simulink model "MicroFSMPCCLACPU1"  (R2024a)
settings: Solver=FixedStepAuto  StartTime=0.0  StopTime=Inf  RelTol=1e-3  EnableMultiTasking=on
values from neighbouring files (symbols this model uses):
  ar = single(round(1/10,3))    [Para_Motor_Micro.m]
  PI_params = mcb.internal.SetControllerParameters(pmsm,inverter,SI_System,T_pwm,Ts,Ts_speed)    [Para_Motor_Micro.m]
  Tabf = round(Tab',3)    [Para_Motor_Micro.m]
  target = mcb_SetProcessorDetails('F28379D',PWM_frequency)    [Para_Motor_Micro.m]
  Ts = T_pwm    (= 3e-05)    [Para_Motor_Micro.m]
  Ts_com = 2*1*Ts    (= 6e-05)    [Para_Motor_Micro.m]
undefined symbols (not defined in the file or in its folder): C28x, codertarget, CPU1, CPU2, Down, dyV, gmax, GPTRIP1SEL, GPTRIP2SEL, inverter, Ls, PWM_Counter_PeriodVel, R, Tab, Tv, Tvz, TZ1, TZ2, ud, Up
libraries: mcbcontrolslib x28, c2802xlib x18, c2837xDlib x13, dsparch4 x6, eeTransforms x5, slpidlib x4, mcbpositiondecoderlib x3, simulink x2, c2806xlib x1, spsabctoAlphaBetaZeroLib x1, c280xlib x1, c2000lib x1
(part 1 of 8)
settings Model: ExtModeTrigDuration=8  Creator=axel_  LastModifiedBy=axel_
settings SolverCC: AutoInsertRateTranBlk=on
settings OptimizationCC: DefaultParameterBehavior=Inlined  DefaultUnderspecifiedDataType=single  EnhancedBackFolding=on  PassReuseOutputArgsAs=Individual arguments  MaxStackSize=1024  OptimizeBlockOrder=speed  DifferentSizesBufferReuse=on  OptimizationCustomize=off  DenormalBehavior=FlushToZero  EfficientTunableParamExpr=on
settings DebuggingCC: MultiTaskDSMMsg=none  ParameterPrecisionLossMsg=none  ParameterTunabilityLossMsg=error
settings HardwareCC: ProdBitPerChar=16  ProdBitPerInt=16  ProdBitPerPointer=32  ProdBitPerSizeT=32  ProdBitPerPtrDiffT=32  ProdLargestAtomicInteger=Integer  ProdLargestAtomicFloat=None  ProdWordSize=16  ProdHWDeviceType=Texas Instruments->C2000
settings ModelReferenceCC: ModelReferenceNumInstancesAllowed=Single
settings SFSimCC: MATLABDynamicMemAlloc=off
settings RTWCC: Description=Embedded Coder  SystemTargetFile=ert.tlc  HardwareBoard=TI Delfino F2837xD  TemplateMakefile=ert_default_tmf  Toolchain=Texas Instruments Code Composer Studio (C2000)  GPUComputeCapability=3.5
settings CodeAppCC: ForceParamTrailComments=on  IgnoreCustomStorageClasses=off  OperatorAnnotations=on  SimulinkDataObjDesc=on  SFDataObjDesc=on  InsertBlockDesc=on
settings ERTTargetCC: CodeReplacementLibrary=TI C28x  ExtModeTransport=4  ExtModeStaticAlloc=on  ExtModeAutomaticAllocSize=off  ExtModeStaticAllocSize=10000  ExtModeMexFile=ext_xcp  ExtModeIntrfLevel=Level2 - Open  InlinedParameterPlacement=NonHierarchical

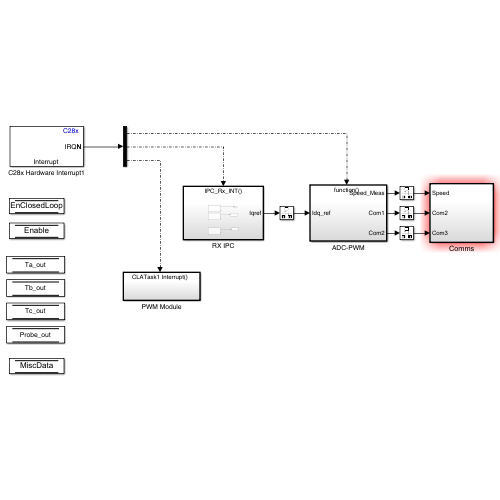
[thumbnail: Simulink's stored preview of the top-level diagram]
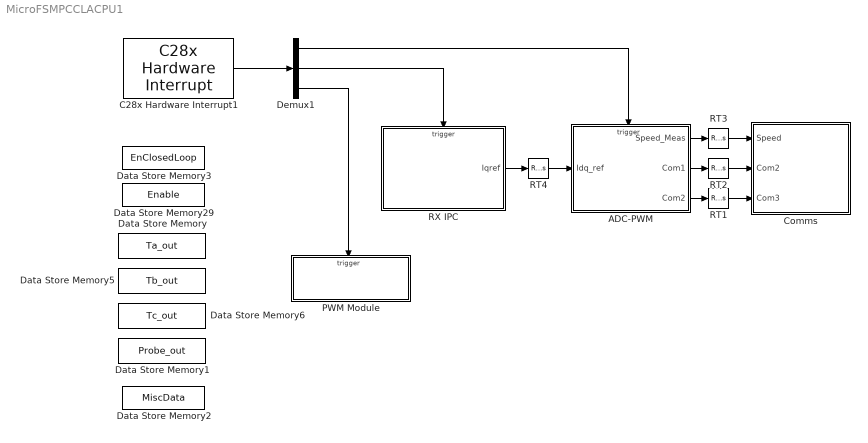
== system MicroFSMPCCLACPU1 ==
  "ADC-PWM " : Subsystem  TreatAsAtomicUnit=on
  C28x Hardware Interrupt1 : c2000lib/Scheduling/C28x Hardware Interrupt  irqnumbers=[1 1 11 ]  pienumbers=[1 15 1 ]  irqpriorities="[30 40  27 ]"  irqpreempts="[1   0  1 ]"  showinput=off  dspchiptype=C280X
  Comms : Subsystem  TreatAsAtomicUnit=on  SystemSampleTime=Ts_com
  Data Store Memory2 : DataStoreMemory  DataStoreName=MiscData  InitialValue=2*pi*0.1296+0.05247  ShowAdditionalParam=off  OutDataTypeStr=single
  Data Store Memory29 : DataStoreMemory  DataStoreName=Enable  ShowAdditionalParam=off  OutDataTypeStr=boolean
  Data Store Memory3 : DataStoreMemory  DataStoreName=EnClosedLoop  ShowAdditionalParam=off  OutDataTypeStr=boolean
  Data Store Memory : DataStoreMemory  DataStoreName=Ta_out  ReadBeforeWriteMsg=warning  WriteAfterWriteMsg=warning  WriteAfterReadMsg=warning  ShowAdditionalParam=off  OutDataTypeStr=single
  Data Store Memory1 : DataStoreMemory  DataStoreName=Probe_out  ReadBeforeWriteMsg=warning  WriteAfterWriteMsg=warning  WriteAfterReadMsg=warning  ShowAdditionalParam=off  OutDataTypeStr=single
  Data Store Memory5 : DataStoreMemory  DataStoreName=Tb_out  ReadBeforeWriteMsg=warning  WriteAfterWriteMsg=warning  WriteAfterReadMsg=warning  ShowAdditionalParam=off  OutDataTypeStr=single
  Data Store Memory6 : DataStoreMemory  DataStoreName=Tc_out  ReadBeforeWriteMsg=warning  WriteAfterWriteMsg=warning  WriteAfterReadMsg=warning  ShowAdditionalParam=off  OutDataTypeStr=single
  Demux1 : Demux  Outputs=3
  PWM Module : Subsystem  TreatAsAtomicUnit=on
  RT{1..4} (4 alike) : RateTransition  Deterministic=off
  RX IPC : Subsystem
  wires:
  C28x Hardware Interrupt1/1 -> Demux1/1
  Demux1/1 -> "ADC-PWM "/Trigger
  "ADC-PWM "/1(Speed_Meas) -> RT3/1
  "ADC-PWM "/2(Com1) -> RT2/1
  "ADC-PWM "/3(Com2) -> RT1/1
  RT3/1 -> Comms/1(Speed)
  RT2/1 -> Comms/2(Com2)
  RT1/1 -> Comms/3(Com3)
  RX IPC/1(Iqref) -> RT4/1
  Demux1/2 -> RX IPC/Trigger
  Demux1/3 -> PWM Module/Trigger
  RT4/1 -> "ADC-PWM "/1(Idq_ref)

== system MicroFSMPCCLACPU1/ADC-PWM  ==
  Idq_ref : Inport
  function : TriggerPort  TriggerType=function-call  VariantControl=Variant  OutputDataType=int8
  Constant : Constant
  Control_System : Subsystem  TreatAsAtomicUnit=on
  Demux1 : Demux  Outputs=2
  Demux2 : Demux  Outputs=2
  Digital Output2 : c2837xDlib/Digital Output  GPIO_Number=GPIO32~GPIO39  GPIO_Bit0=off  GPIO_BIT0_Toggle=on  GPIO_Bit1=off  GPIO_BIT1_Toggle=off  GPIO_Bit2=off  GPIO_BIT2_Toggle=off  GPIO_Bit3=off  GPIO_BIT3_Toggle=off  GPIO_Bit4=off  GPIO_BIT4_Toggle=off  GPIO_Bit5=off  GPIO_BIT5_Toggle=off  GPIO_Bit6=off  GPIO_BIT6_Toggle=off  GPIO_Bit7=on  GPIO_BIT7_Toggle=on
  Mesurments : Subsystem
  Speed_Meas : Outport
  Com1 : Outport  Port=2
  Com2 : Outport  Port=3
  wires:
  Idq_ref/1 -> Control_System/3(Tref)
  Mesurments/1(I) -> Control_System/1(Imesure)
  Mesurments/5(Thetae) -> Control_System/4(PosE)
  Mesurments/2(Voltage Bus) -> Control_System/2(Voltage Bus)
  Control_System/2(Debug control 2) -> Demux1/1
  Constant/1 -> Digital Output2/1
  Mesurments/6(Speedencoder) -> Speed_Meas/1, Control_System/5(Speed)
  Control_System/1(Debug control) -> Demux2/1
  Demux2/2 -> Com2/1
  Demux1/2 -> Com1/1

== system MicroFSMPCCLACPU1/Comms ==
  note: Comms
  Speed : Inport
  Com2 : Inport  Port=2
  Com3 : Inport  Port=3
  Data Store Read2 : DataStoreRead  DataStoreName=EnClosedLoop  IndexOptions=Index vector (dialog)  Indices=1  OutputSizes=1
  Get_ADC_Volt1 : Gain  OutDataTypeStr=single  RndMeth=Simplest
  Get_ADC_Volt6 : Gain  OutDataTypeStr=single  RndMeth=Simplest
  Get_ADC_Volt9 : Gain  OutDataTypeStr=single  RndMeth=Simplest
  IPC Transmit : c2837xDlib/IPC Transmit  blkParamProc=F2837x  SelectDestination=C28x (CPU1/CPU2)  SelectChannel=0  EnableBlocking=off
  IPC Transmit1 : c2837xDlib/IPC Transmit  blkParamProc=F2837x  SelectDestination=C28x (CPU1/CPU2)  SelectChannel=1  EnableBlocking=off
  IPC Transmit2 : c2837xDlib/IPC Transmit  blkParamProc=F2837x  SelectDestination=C28x (CPU1/CPU2)  SelectChannel=4  EnableBlocking=off
  Mux : Mux  Inputs=2
  wires:
  Speed/1 -> Get_ADC_Volt9/1
  Com2/1 -> Get_ADC_Volt6/1
  Get_ADC_Volt9/1 -> IPC Transmit/1
  Com3/1 -> Get_ADC_Volt1/1
  Get_ADC_Volt6/1 -> Mux/1
  Get_ADC_Volt1/1 -> Mux/2
  Mux/1 -> IPC Transmit1/1
  Data Store Read2/1 -> IPC Transmit2/1

== system MicroFSMPCCLACPU1/PWM Module ==
  CLATask1 Interrupt : TriggerPort  TriggerType=function-call  VariantControl=Variant
  Constant : Constant
  Data Store Read : DataStoreRead  DataStoreName=Ta_out  IndexOptions=Index vector (dialog)  Indices=1  OutputSizes=1
  Data Store Read1 : DataStoreRead  DataStoreName=Tb_out  IndexOptions=Index vector (dialog)  Indices=1  OutputSizes=1
  Data Store Read2 : DataStoreRead  DataStoreName=Tc_out  IndexOptions=Index vector (dialog)  Indices=1  OutputSizes=1
  Digital Output1 : c2837xDlib/Digital Output  GPIO_Number=GPIO16~GPIO23  GPIO_Bit0=off  GPIO_BIT0_Toggle=on  GPIO_Bit1=off  GPIO_BIT1_Toggle=off  GPIO_Bit2=off  GPIO_BIT2_Toggle=off  GPIO_Bit3=off  GPIO_BIT3_Toggle=off  GPIO_Bit4=off  GPIO_BIT4_Toggle=off  GPIO_Bit5=off  GPIO_BIT5_Toggle=off  GPIO_Bit6=on  GPIO_BIT6_Toggle=on  GPIO_Bit7=off  GPIO_BIT7_Toggle=off
  Enable1 : DataStoreRead  DataStoreName=Enable  IndexOptions=Index vector (dialog)  Indices=1  OutputSizes=1
  Inverter (Code Generation) : Subsystem
  Mux : Mux  Inputs=3
  Mux8 : Mux  Inputs=2
  ata Type Conversion1 : DataTypeConversion  OutDataTypeStr=single  SaturateOnIntegerOverflow=off  RndMeth=Floor
  wires:
  Data Store Read/1 -> Mux/1
  Data Store Read1/1 -> Mux/2
  Data Store Read2/1 -> Mux/3
  Mux/1 -> Mux8/1
  ata Type Conversion1/1 -> Mux8/2
  Enable1/1 -> ata Type Conversion1/1
  Mux8/1 -> Inverter (Code Generation)/1(Inverter Signals)
  Constant/1 -> Digital Output1/1

== system MicroFSMPCCLACPU1/RX IPC ==
  note: Data 1
  note: Te
  IPC_Rx_INT : TriggerPort  TriggerType=function-call  VariantControl=Variant
  Data Store Write : DataStoreWrite  DataStoreName=Enable  IndexOptions=Index vector (dialog)  Indices=1  OutputSizes=1
  Data Store Write1 : DataStoreWrite  DataStoreName=MiscData  IndexOptions=Index vector (dialog)  Indices=1  OutputSizes=1
  IPC Receive1 : c2837xDlib/IPC Receive  blkParamProc=F2837x  SelectSource=C28x (CPU1/CPU2)  SelectChannel=2  DataType=single  DataLength=1  EnableBlocking=off  SampleTime=-1
  IPC Receive2 : c2837xDlib/IPC Receive  blkParamProc=F2837x  SelectSource=C28x (CPU1/CPU2)  SelectChannel=3  DataType=boolean  DataLength=1  EnableBlocking=off  SampleTime=-1
  IPC Receive3 : c2837xDlib/IPC Receive  blkParamProc=F2837x  SelectSource=C28x (CPU1/CPU2)  SelectChannel=5  DataType=single  DataLength=1  EnableBlocking=off  SampleTime=-1
  Iqref : Outport
  wires:
  IPC Receive1/1 -> Iqref/1
  IPC Receive2/1 -> Data Store Write/1
  IPC Receive3/1 -> Data Store Write1/1

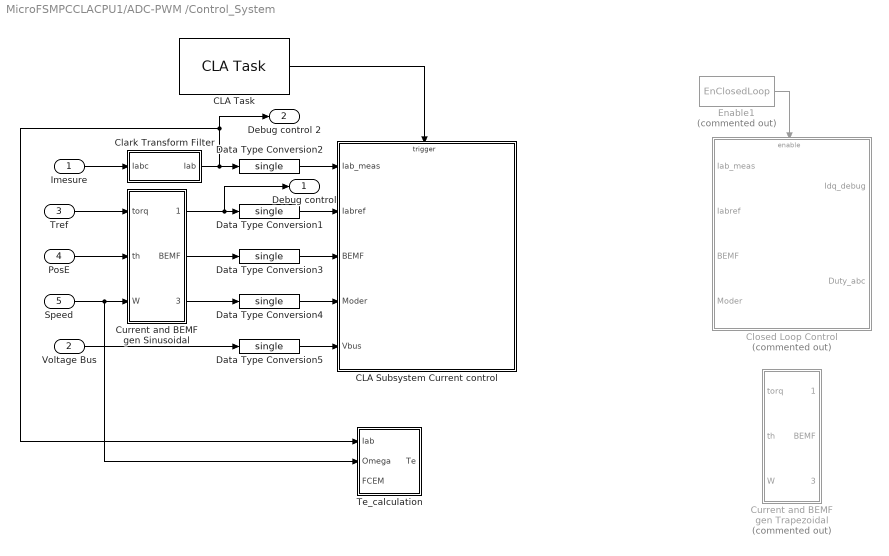
== system MicroFSMPCCLACPU1/ADC-PWM /Control_System ==
  Imesure : Inport
  Voltage Bus : Inport  Port=2
  Tref : Inport  Port=3
  PosE : Inport  Port=4
  Speed : Inport  Port=5
  CLA Subsystem Current control : Subsystem  InitFcn=codertarget.registry.registerC28xNonPeripheralBlocks(gcb)  TreatAsAtomicUnit=on  RTWFileName=sample_cla  mask(c28x CLA Subsystem){clasubsystem=1}
      mask prompts: clasubsystem "CLA Subsystem"
      mask help: A CLA Subsystem template containing an input and outport block.
      settings: LibrarySourceBlock=c2837xDlib/CLA Subsystem  CopyFcn=codertarget.registry.setC28xCLASubSystem(gcb)  OpenFcn=open_system(gcbh,'force')  RTWSystemCode=Nonreusable function  RTWFileNameOpts=User specified  FunctionWithSeparateData=on  RTWMemSecFuncInitTerm=C28xFunction  RTWMemSecFuncExecute=ClaFunction  RTWMemSecDataConstants=Cla1DataRam  RTWMemSecDataInternal=Cla1DataRam  RTWMemSecDataParameters=Cla1DataRam
      mask Help: eval('codertarget.internal.helpView(''tic2000'' ,''c28xCLASubsystem'')')
      mask Display: color('black'); text(0.50, 0.12, 'CLA Subsystem', 'horizontalAlignment','center');
  CLA Task : c2806xlib/CLA Task  taskNumber=1  intSource=Software  wait=off  sampleTime=-1  claType=1  softTrigSelected=1  enableInterrupt=on
      settings: LibrarySourceBlock=c2837xDlib/CLA Task
  Clark Transform Filter : Subsystem
  Closed Loop Control : Subsystem  Commented=on
  Current and BEMF gen Sinusoidal : Subsystem
  Current and BEMF gen Trapezoidal : Subsystem  Commented=on
  Data Type Conversion{1..5} (5 alike) : DataTypeConversion  OutDataTypeStr=single  SaturateOnIntegerOverflow=off  RndMeth=Floor
  Enable1 : DataStoreRead  Commented=on  DataStoreName=EnClosedLoop  IndexOptions=Index vector (dialog)  Indices=1  OutputSizes=1
  Te_calculation : Subsystem
  Debug control : Outport
  Debug control 2 : Outport  Port=2
  wires:
  Imesure/1 -> Clark Transform Filter/1(Iabc)
  Current and BEMF gen Sinusoidal/1(Iabref) -> Debug control/1, Data Type Conversion1/1
  Current and BEMF gen Sinusoidal/2(BEMF) -> Data Type Conversion3/1
  Current and BEMF gen Sinusoidal/3(Moder) -> Data Type Conversion4/1
  CLA Task/1 -> CLA Subsystem Current control/Trigger
  Enable1/1 -> Closed Loop Control/Enable
  Tref/1 -> Current and BEMF gen Sinusoidal/1(torq)
  PosE/1 -> Current and BEMF gen Sinusoidal/2(th)
  Speed/1 -> Te_calculation/2(Omega), Current and BEMF gen Sinusoidal/3(W)
  Data Type Conversion2/1 -> CLA Subsystem Current control/1(Iab_meas)
  Data Type Conversion1/1 -> CLA Subsystem Current control/2(Iabref)
  Data Type Conversion3/1 -> CLA Subsystem Current control/3(BEMF)
  Data Type Conversion4/1 -> CLA Subsystem Current control/4(Moder)
  Clark Transform Filter/1(Iab) -> Te_calculation/1(Iab), Debug control 2/1, Data Type Conversion2/1
  Voltage Bus/1 -> Data Type Conversion5/1
  Data Type Conversion5/1 -> CLA Subsystem Current control/5(Vbus)

== system MicroFSMPCCLACPU1/ADC-PWM /Mesurments ==
  Current mesurment : Subsystem
  Position Mesurment : Subsystem
  Voltage Mesurment : Subsystem
  I : Outport
  Voltage Bus : Outport  Port=2
  Voltage : Outport  Port=3
  ThetaMec : Outport  Port=4
  Thetae : Outport  Port=5
  Speedencoder : Outport  Port=6
  wires:
  Current mesurment/1(Out1) -> I/1
  Voltage Mesurment/1(Out1) -> Voltage Bus/1
  Voltage Mesurment/2(Vol) -> Voltage/1
  Position Mesurment/1(ThetaE) -> Thetae/1
  Position Mesurment/3(ThetaMec) -> ThetaMec/1
  Position Mesurment/2(speedfb) -> Speedencoder/1
